simulink model "main"  (R2019b)
settings: Solver=FixedStepAuto  StartTime=0.0  StopTime=7199  FixedStep=1  RelTol=1e-3
libraries: fuzblock x1, powerlib_meascontrol x1
settings Model: Creator=hfekriaz  LastModifiedBy=hfekriaz

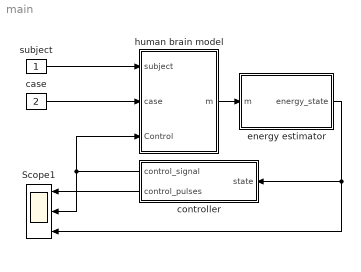
== system main ==
  Scope1 : Scope  NumInputPorts=3
  case : Constant  Value=2
  controller : Subsystem
  energy estimator : Subsystem
  human brain model : Subsystem
  "subject " : Constant
  wires:
  energy estimator/1(energy_state) -> Scope1/3, controller/1(state)
  human brain model/1(m) -> energy estimator/1(m)
  controller/2(control_pulses) -> Scope1/1
  controller/1(control_signal) -> human brain model/3(Control), Scope1/2
  "subject "/1 -> human brain model/1(subject)
  case/1 -> human brain model/2(case)

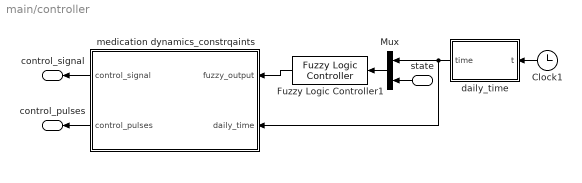
== system main/controller ==
  state : Inport
  Clock1 : Clock
      settings: Decimation=10000
  Fuzzy Logic Controller1 : fuzblock/Fuzzy Logic  Controller  FIS='fuzzy_sys.fis'  OutputSampleNumber=101  DataType=double  FuzzifiedInputs=off  RuleFiringStrengths=off  RuleOutputs=off  AggregatedOutputs=off  SimulateUsing=Interpreted execution  OutOfRangeInputValueMessage=warning  NoRuleFiredMessage=warning  EmptyOutputFuzzySetMessage=warning
  Mux : Mux  Inputs=2
  daily_time : MATLAB Function  TreatAsAtomicUnit=on
  "medication dynamics_constrqaints " : Subsystem
  control_signal : Outport  VectorParamsAs1DForOutWhenUnconnected=off
  control_pulses : Outport  Port=2  VectorParamsAs1DForOutWhenUnconnected=off
  wires:
  Clock1/1 -> daily_time/1(t)
  daily_time/1(time) -> "medication dynamics_constrqaints "/2(daily_time), Mux/1
  state/1 -> Mux/2
  Mux/1 -> Fuzzy Logic Controller1/1
  Fuzzy Logic Controller1/1 -> "medication dynamics_constrqaints "/1(fuzzy_output)
  "medication dynamics_constrqaints "/2(control_pulses) -> control_pulses/1
  "medication dynamics_constrqaints "/1(control_signal) -> control_signal/1

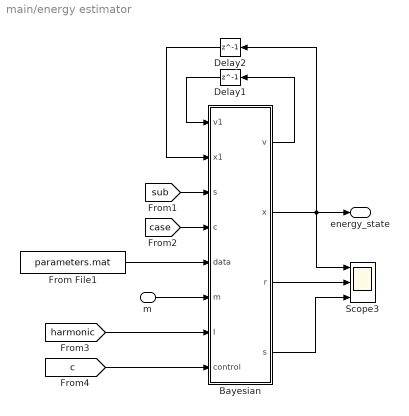
== system main/energy estimator ==
  m : Inport
  Bayesian : MATLAB Function  TreatAsAtomicUnit=on
  Delay1 : Delay  DelayLength=1  InitialCondition=0.0038
  Delay2 : Delay  DelayLength=1  InitialCondition=0.21932
  From File1 : FromFile  FileName=parameters.mat
  Scope3 : Scope  NumInputPorts=3
  energy_state : Outport  VectorParamsAs1DForOutWhenUnconnected=off
  wires:
  From File1/1 -> Bayesian/5(data)
  Delay2/1 -> Bayesian/2(x1)
  Delay1/1 -> Bayesian/1(v1)
  m/1 -> Bayesian/6(m)
  Bayesian/1(v) -> Delay1/1
  [sub] -> Bayesian/3("s ")
  [case] -> Bayesian/4(c)
  [harmonic] -> Bayesian/7(I)
  [c] -> Bayesian/8(control)
  Bayesian/2(x) -> Scope3/1, energy_state/1, Delay2/1
  Bayesian/3(r) -> Scope3/2
  Bayesian/4(s) -> Scope3/3

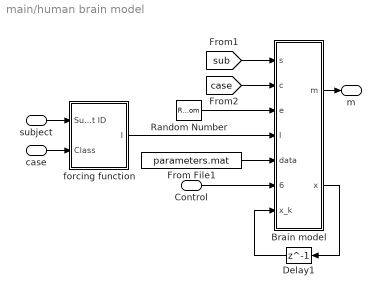
== system main/human brain model ==
  subject : Inport
  case : Inport  Port=2
  Control : Inport  Port=3
  Brain model : MATLAB Function  TreatAsAtomicUnit=on
  Delay1 : Delay  DelayLength=1  InitialCondition=0.21932
  From File1 : FromFile  FileName=parameters.mat
  Random Number : RandomNumber  Variance=0.0103  Seed=50  SampleTime=1
  "forcing function " : Subsystem
  m : Outport  VectorParamsAs1DForOutWhenUnconnected=off
  wires:
  [sub] -> Brain model/1(s)
  From File1/1 -> Brain model/5(data)
  Delay1/1 -> Brain model/7(x_k)
  Brain model/2(x) -> Delay1/1
  Random Number/1 -> Brain model/3(e)
  Brain model/1(m) -> m/1
  Control/1 -> Brain model/6(control)
  [case] -> Brain model/2(c)
  "forcing function "/1(I) -> Brain model/4(I)
  case/1 -> "forcing function "/2(Class)
  subject/1 -> "forcing function "/1(Subject ID)

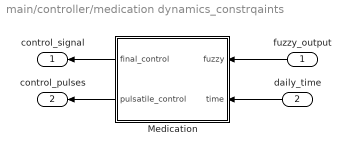
== system main/controller/medication dynamics_constrqaints  ==
  fuzzy_output : Inport
  daily_time : Inport  Port=2
  Medication : Subsystem
  control_signal : Outport  VectorParamsAs1DForOutWhenUnconnected=off
  control_pulses : Outport  Port=2  VectorParamsAs1DForOutWhenUnconnected=off
  wires:
  fuzzy_output/1 -> Medication/1(fuzzy)
  daily_time/1 -> Medication/2(time)
  Medication/1(final_control) -> control_signal/1
  Medication/2(pulsatile_control) -> control_pulses/1

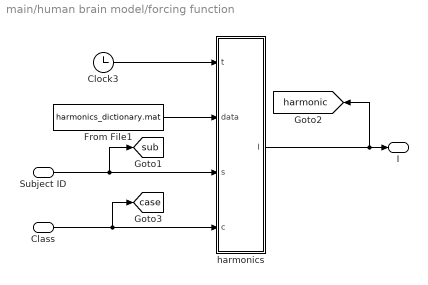
== system main/human brain model/forcing function  ==
  Subject ID : Inport
  Class : Inport  Port=2
  Clock3 : Clock
      settings: Decimation=10000
  From File1 : FromFile  FileName=harmonics_dictionary.mat
  harmonics : MATLAB Function  TreatAsAtomicUnit=on
  I : Outport  VectorParamsAs1DForOutWhenUnconnected=off
  tag scope: case=global, harmonic=global, sub=global
  wires:
  Clock3/1 -> harmonics/1(t)
  From File1/1 -> harmonics/2(data)
  harmonics/1(I) -> [harmonic], I/1
  Subject ID/1 -> [sub], harmonics/3(s)
  Class/1 -> [case], harmonics/4(c)

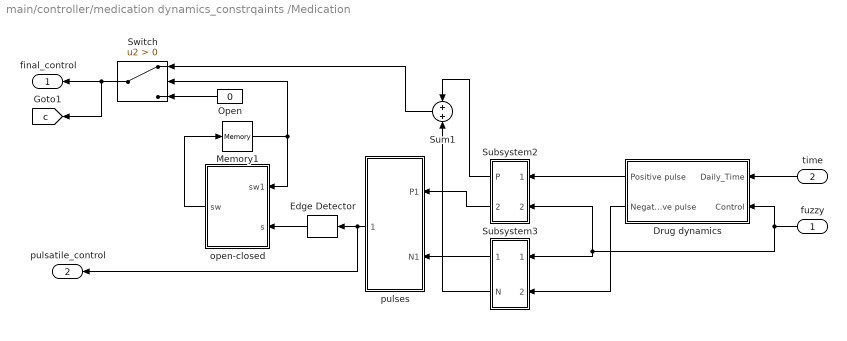
== system main/controller/medication dynamics_constrqaints /Medication ==
  fuzzy : Inport
  time : Inport  Port=2
  Drug dynamics : Subsystem
  Edge Detector : powerlib_meascontrol/Logic/Edge Detector  model=Rising  ic=0  Ts=0
      settings: SourceProductName=Simscape Electrical  SourceProductBaseCode=PS
  Memory1 : Memory
  Open : Constant  Value=0
  Subsystem2 : Subsystem
  Subsystem3 : Subsystem
  Sum1 : Sum
  Switch : Switch  Criteria=u2 > Threshold
  open-closed : MATLAB Function  TreatAsAtomicUnit=on
  pulses : Subsystem
  final_control : Outport  VectorParamsAs1DForOutWhenUnconnected=off
  pulsatile_control : Outport  Port=2  VectorParamsAs1DForOutWhenUnconnected=off
  tag scope: c=global
  wires:
  Subsystem2/2(P1) -> pulses/1(P1)
  Subsystem3/1(N1) -> pulses/2(N1)
  Drug dynamics/2("Negative pulse ") -> Subsystem3/2(Tn)
  fuzzy/1 -> Drug dynamics/2(Control), Subsystem2/2(Cp), Subsystem3/1(Cn)
  time/1 -> Drug dynamics/1(Daily_Time)
  Drug dynamics/1("Positive pulse ") -> Subsystem2/1(Tp)
  pulses/1(pulse_control) -> pulsatile_control/1, Edge Detector/1
  Edge Detector/1 -> open-closed/2(s)
  Memory1/1 -> open-closed/1(sw1), Switch/2
  open-closed/1(sw) -> Memory1/1
  Switch/1 -> final_control/1, [c]
  Sum1/1 -> Switch/1
  Open/1 -> Switch/3
  Subsystem2/1(P) -> Sum1/1
  Subsystem3/2("N ") -> Sum1/2

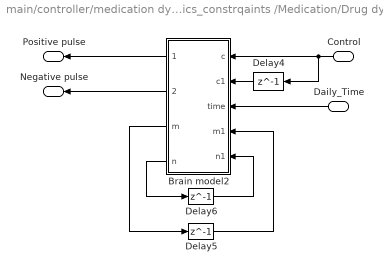
== system main/controller/medication dynamics_constrqaints /Medication/Drug dynamics ==
  Daily_Time : Inport
  Control : Inport  Port=2
  Brain model2 : MATLAB Function  TreatAsAtomicUnit=on
  Delay4 : Delay  DelayLength=1  InitialCondition=0
  Delay5 : Delay  DelayLength=1  InitialCondition=0
  Delay6 : Delay  DelayLength=1  InitialCondition=0
  "Positive pulse " : Outport  VectorParamsAs1DForOutWhenUnconnected=off
  "Negative pulse " : Outport  Port=2  VectorParamsAs1DForOutWhenUnconnected=off
  wires:
  Brain model2/1(control_p) -> "Positive pulse "/1
  Control/1 -> Delay4/1, Brain model2/1(c)
  Delay5/1 -> Brain model2/4(m1)
  Delay4/1 -> Brain model2/2(c1)
  Brain model2/3(m) -> Delay5/1
  Delay6/1 -> Brain model2/5(n1)
  Daily_Time/1 -> Brain model2/3(time)
  Brain model2/4(n) -> Delay6/1
  Brain model2/2(control_n) -> "Negative pulse "/1

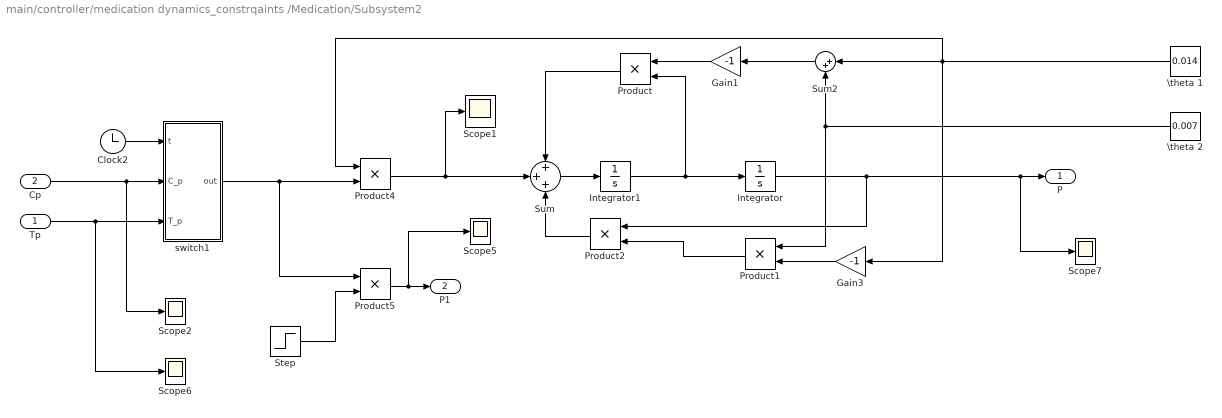
== system main/controller/medication dynamics_constrqaints /Medication/Subsystem2 ==
  Tp : Inport
  Cp : Inport  Port=2
  Clock2 : Clock
      settings: Decimation=10000
  Gain1 : Gain  Gain=-1
  Gain3 : Gain  Gain=-1
  Integrator : Integrator
  Integrator1 : Integrator
  Product{,1..2,4..5} (5 alike) : Product
  Scope{1..2,5..7} (5 alike) : Scope
  Step : Step  Time=2880  SampleTime=0
  Sum : Sum  Inputs=+++
  Sum2 : Sum  Inputs=|++
  \theta 1 : Constant  Value=0.014
  \theta 2 : Constant  Value=0.007
  switch1 : MATLAB Function  TreatAsAtomicUnit=on
  P : Outport  VectorParamsAs1DForOutWhenUnconnected=off
  P1 : Outport  Port=2  VectorParamsAs1DForOutWhenUnconnected=off
  wires:
  Sum2/1 -> Gain1/1
  Product4/1 -> Scope1/1, Sum/2
  Product1/1 -> Product2/2
  Product2/1 -> Sum/3
  \theta 1/1 -> Product4/1, Sum2/1, Gain3/1
  Integrator1/1 -> Product/2, Integrator/1
  Integrator/1 -> Product2/1, Scope7/1, P/1
  Product/1 -> Sum/1
  \theta 2/1 -> Product1/1, Sum2/2
  Sum/1 -> Integrator1/1
  Gain1/1 -> Product/1
  Gain3/1 -> Product1/2
  switch1/1(out) -> Product5/1, Product4/2
  Clock2/1 -> switch1/1(t)
  Cp/1 -> Scope2/1, switch1/2(C_p)
  Tp/1 -> Scope6/1, switch1/3(T_p)
  Product5/1 -> Scope5/1, P1/1
  Step/1 -> Product5/2

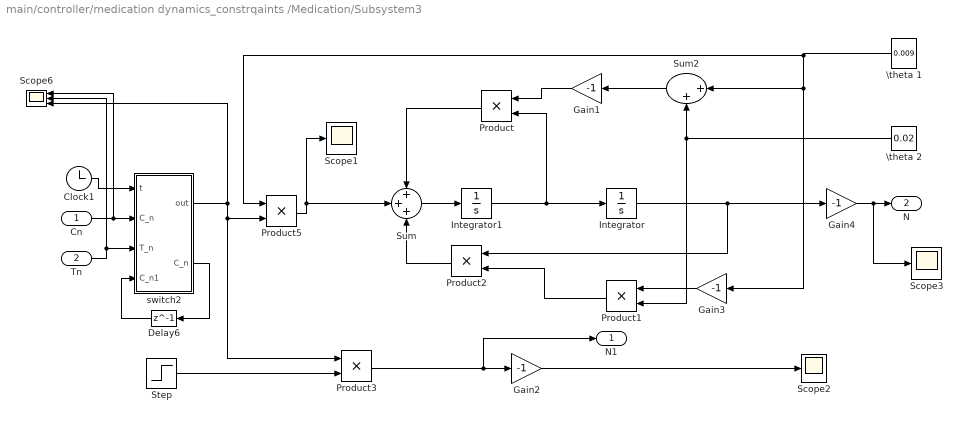
== system main/controller/medication dynamics_constrqaints /Medication/Subsystem3 ==
  Cn : Inport
  Tn : Inport  Port=2
  Clock1 : Clock
      settings: Decimation=10000
  Delay6 : Delay  DelayLength=1  InitialCondition=0
  Gain{1..4} (4 alike) : Gain  Gain=-1
  Integrator : Integrator
  Integrator1 : Integrator  InitialCondition=0.00001
  Product{,1..3,5} (5 alike) : Product
  Scope1 : Scope
  Scope2 : Scope
  Scope3 : Scope
  Scope6 : Scope  NumInputPorts=3
  Step : Step  Time=2880  SampleTime=0
  Sum : Sum  Inputs=+++
  Sum2 : Sum  Inputs=|++
  \theta 1 : Constant  Value=0.009
  \theta 2 : Constant  Value=0.02
  switch2 : MATLAB Function  TreatAsAtomicUnit=on
  N1 : Outport  VectorParamsAs1DForOutWhenUnconnected=off
  "N " : Outport  Port=2  VectorParamsAs1DForOutWhenUnconnected=off
  wires:
  Gain1/1 -> Product/1
  Sum/1 -> Integrator1/1
  \theta 2/1 -> Sum2/2, Product1/2
  Gain3/1 -> Product1/1
  Product/1 -> Sum/1
  Integrator/1 -> Gain4/1, Product2/1
  Integrator1/1 -> Integrator/1, Product/2
  Product2/1 -> Sum/3
  Product1/1 -> Product2/2
  Product5/1 -> Sum/2, Scope1/1
  Sum2/1 -> Gain1/1
  Gain4/1 -> Scope3/1, "N "/1
  \theta 1/1 -> Gain3/1, Sum2/1, Product5/1
  Cn/1 -> Scope6/1, switch2/2("C_n ")
  Clock1/1 -> switch2/1(t)
  Tn/1 -> Scope6/2, switch2/3(T_n)
  switch2/1(out) -> Product3/1, Product5/2, Scope6/3
  Product3/1 -> Gain2/1, N1/1
  Step/1 -> Product3/2
  Gain2/1 -> Scope2/1
  switch2/2(C_n) -> Delay6/1
  Delay6/1 -> switch2/4(C_n1)

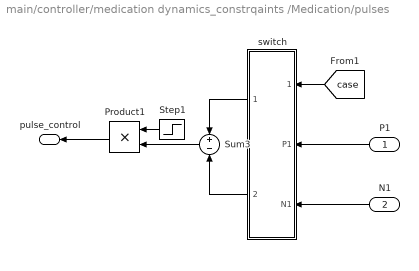
== system main/controller/medication dynamics_constrqaints /Medication/pulses ==
  P1 : Inport
  N1 : Inport  Port=2
  Product1 : Product
  Step1 : Step  Time=2880  SampleTime=0
  Sum3 : Sum  Inputs=+-
  switch : MATLAB Function  TreatAsAtomicUnit=on
  pulse_control : Outport  VectorParamsAs1DForOutWhenUnconnected=off
  wires:
  Sum3/1 -> Product1/2
  [case] -> switch/1(class)
  switch/1(pulse_p) -> Sum3/1
  Step1/1 -> Product1/1
  switch/2(pulse_n) -> Sum3/2
  P1/1 -> switch/2(P1)
  N1/1 -> switch/3(N1)
  Product1/1 -> pulse_control/1

== matlab function main/controller/medication dynamics_constrqaints /Medication/pulses/switch ==
  data: class input; P1 input; N1 input; pulse_p output; pulse_n output
function [pulse_p,pulse_n]  = fcn(class,P1,N1)

if class == 1
    pulse_p = 0;
    pulse_n = 0;
else
    pulse_p = P1;
    pulse_n = N1;
end
end

== matlab function main/controller/medication dynamics_constrqaints /Medication/open-closed ==
  data: sw1 input; s input; sw output
function sw  = fcn(sw1,s)

sw = s + sw1;


end

== matlab function main/energy estimator/Bayesian ==
  settings: updateMethod=DISCRETE
  data: v1 input; x1 input; s input; c input; data input; v output; x output; m input; I input; r output; s output; control input
function [v,x,r,s]=fcn(v1,x1,s,c,data,m,I,control)
i = 3*(s-1) + c;
param = data(11*(i-1)+1:11*(i));  %%%% using the estimated model parametrs as a results of oofline EM algorithm 

%%% make sure to use the corresponding model parametrs in the initial condittion x_0 and v_0

% param(---,:) = 
% 1-[x0 ;
% 2-ve ;
% 3-rho ;
% 4-r0 ;
% 5-r1 ;
% 6-vr ;
% 7-s0 ;
% 8-s1 ;
% 9-vs ;
% 10-b0 ;
% 11-b1 ]

beta_0 =  param(10);
beta_1 =  param(11);
vs =  param(9);
s1 =  param(8);
s0 =  param(7);
vr =  param(6);
r1 =  param(5);
r0 =  param(4);
rho = param(3);
ve =  param(2);
x0 = param(1);

v0 = ve;
x_upd = rho*x1 + I +control;
v_upd = (rho ^ 2) *v1 + ve;

%%%%
r = normrnd(r0 + r1*x_upd,vr^0.5);
s = normrnd(s0 + s1*x_upd,vs^0.5);
C = v_upd / (vr * vs + v_upd * ((r1 ^ 2) * vs + (s1 ^ 2) * vr));

M = 200;
it = zeros(1, M);
f = zeros(1, M);
df = zeros(1, M);

% y = NaN;
it(1) = x_upd;
sol = 0;
for i = 1:(M - 1)
    f(i) = it(i) - x_upd - C * (r1 * vs * (r - r0 - r1 * x_upd) + s1 * vr * (s - s0 - s1 * x_upd) + ...
        vr * vs * beta_1 * (m - (1 / (1 + exp((-1) * (beta_0 + beta_1 * it(i))))))); 
    df(i) = 1 + C * vr * vs * (beta_1 ^ 2) * exp(beta_0 + beta_1 * it(i)) / ((1 + exp(beta_0 + beta_1 * it(i))) ^ 2);
    it(i + 1) = it(i) - f(i) / df(i);
    sol = it(i + 1) ;
    if abs(sol - it(i)) > 1e-14
        continue 
    end
end

x = sol;
p = 1 / (1 + exp((-1) * (beta_0 + beta_1 * x)));
v = 1 / ((1 / v_upd) + ((r1 ^ 2) / vr) + ((s1 ^ 2) / vs) + (beta_1 ^ 2) * p * (1 - p));        
end

== matlab function main/human brain model/Brain model ==
  settings: updateMethod=DISCRETE
  data: s input; c input; e input; I input; data input; control input; m output; x output; x_k input
function [m,x] = fcn(s,c,e,I, data,control,x_k)
i = 3*(s-1) + c;
param = data(11*(i-1)+1:11*(i)); %%%% using the estimated model parametrs as a results of oofline EM algorithm 

%%% make sure to use the corresponding model parametrs in the initial condittion x_0

% param(---,:) = 
% 1-[x0 ;
% 2-ve ;
% 3-rho ;
% 4-r0 ;
% 5-r1 ;
% 6-vr ;
% 7-s0 ;
% 8-s1 ;
% 9-vs ;
% 10-b0 ;
% 11-b1 ]

x0 =param(1) ;
rho = param(3);
beta_0 =  param(10);
beta_1 =  param(11);

x = rho*x_k + control + I + e ; %control includes I as well 

p = 1/(1+exp(-1*(beta_1*x + beta_0))); %sigmoid function
m=0;
if rand(1)<p
    m = 1;
end

end

== matlab function main/controller/medication dynamics_constrqaints /Medication/Subsystem2/switch1 ==
  data: out output; t input; C_p input; T_p input
function out  = fcn(t,C_p,T_p)
T = 1440; 
n = floor(t/T);

cc =  0;


if T_p >0
%  if  t > T_p + n*T && t< T_p + 3 + n*T
    cc  = 1;
else 
    cc = 0 ;
end

out = C_p*cc;


end

== matlab function main/controller/medication dynamics_constrqaints /Medication/Subsystem3/switch2 ==
  data: out output; t input; C_n input; T_n input; C_n output; C_n1 input
function [out,C_n]  = fcn(t,C_n,T_n,C_n1)
T = 1440; 
n = floor(t/T);
% control = C_n - C_n1;%%%%%%%%
cc =  0;
if T_n >0
% if  t == T_n + n*T 
% if  t > T_n + n*T && t< T_n + 2  + n*T
    cc  = 1;
else 
    cc = 0 ;
end
if C_n <0
    
    C_n = -1*C_n;
    C_n1 = -1*C_n1;
    
end 
% out = C_n*cc;
out = (C_n - C_n1)*cc;


end

== matlab function main/controller/medication dynamics_constrqaints /Medication/Drug dynamics/Brain model2 ==
  settings: updateMethod=DISCRETE
  data: control_p output; control_n output; m output; n output; c input; c1 input; time input; m1 input; n1 input
function [control_p,control_n,m,n] = fcn(c,c1,time,m1,n1)
c_time = c-c1;
control = c_time;
x = control;
y = control;

%%% Negative pulses

control_n = 0;
if y > - 0.01
    y = 0;
end

if y<0 && time > 17 %%%% 12 for sub = 5  and 17 for others 
    n = n1+1;
    control_n = c;
else
    n = n1+ 0 ;
end

if n > 1 && time < 23.97 
    control_n = 0;
end
control_n = -1*control_n;

%%% Postive pulses

control_p = 0 ;    

if x<0.016
    x = 0;
end

if x>0 &&  time < 17
    m = m1+1;
    control_p = c;
else
    m = m1 + 0;
end

if m > 1 && time < 23.97 
    control_p = 0;
end


if time > 23.97
   m = 0;
   n=0;
end

end

== matlab function main/controller/daily_time ==
  data: time output; t input
function time    = fcn(t)
T_day = 1440; 

T_s = floor(t/T_day)*T_day; 
time = t - T_s;
time = time /60;
end

== matlab function main/human brain model/forcing function /harmonics ==
  data: t input; data input; s input; c input; I output
function I = fcn(t,data,s,c)

T = 1440;

%%% Directory for the harmonic function I_k
i = 3*(s-1) + c;  %%% s: subject (1:10) , c:class (1:3)
param = data(5*(i-1)+1:5*(i));
    % param(---,:) = 
    % 1-[a0 ;
    % 2-a1 ;
    % 3-b1 ;
    % 4-a2 ;
    % 5-b2 ;]

a0 = param(1); a1 = param(2); b1 = param(3); a2 = param(4); b2 = param(5);
  
I = a0 + a1 * sin(2 * pi * t / T) + b1 * cos(2 * pi * t / T) + ...
        a2 * sin(2 * pi * t / (T / 2)) + b2 * cos(2 * pi * t / (T / 2));

end
